simulink model "es"  (Simulink 8.3)
settings: Solver=ode45  StartTime=0.0  StopTime=20  RelTol=1e-3
values from neighbouring files (symbols this model uses):
  D1 = 1    [es.m]
  Kr = 1    [es.m]
libraries: cstblocks x2
settings Model: Creator=matdo  LastModifiedBy=matdo
settings DataIOCC: SignalLoggingSaveFormat=Dataset
settings DebuggingCC: UnderspecifiedInitializationDetection=Simplified  StateNameClashWarn=none
settings GRTTargetCC: CombineOutputUpdateFcns=on  GRTInterface=off

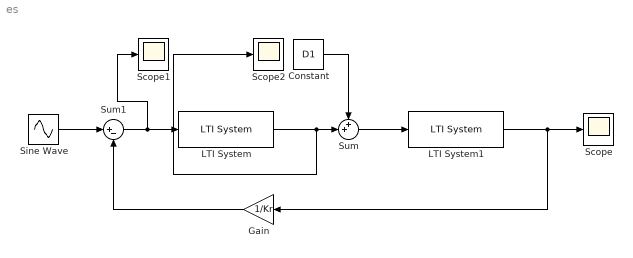
== system es ==
  Constant : Constant  Value=D1
  Gain : Gain  Gain=1/Kr
  LTI System : cstblocks/LTI System  sys=Ci  IC=[]
  LTI System1 : cstblocks/LTI System  sys=F  IC=[]
  Scope : Scope
  Scope1 : Scope
  Scope2 : Scope
      settings: SaveName=ScopeData2
  Sine Wave : Sin  Frequency=0.1  SampleTime=0
  Sum : Sum  Inputs=++|
  Sum1 : Sum  Inputs=|+-
  wires:
  Constant/1 -> Sum/1
  LTI System/1 -> Scope2/1, Sum/2
  Sum/1 -> LTI System1/1
  Sine Wave/1 -> Sum1/1
  Gain/1 -> Sum1/2
  Sum1/1 -> Scope1/1, LTI System/1
  LTI System1/1 -> Gain/1, Scope/1
